simulink model "Check_predictblock"  (R2025b)
settings: Solver=FixedStepAuto  StartTime=0.0  StopTime=1  FixedStep=1/135  RelTol=1e-3
libraries: deeplib x1
settings Model: Creator=faizshaikh  LastModifiedBy=faizshaikh

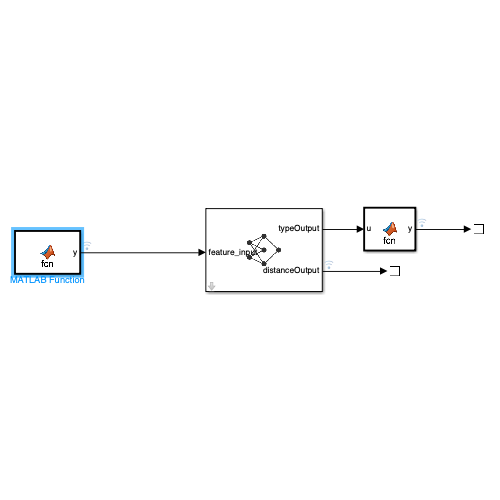
[thumbnail: Simulink's stored preview of the top-level diagram]
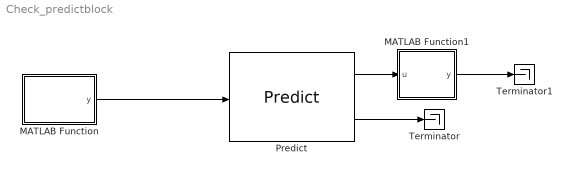
== system Check_predictblock ==
  MATLAB Function : MATLAB Function  TreatAsAtomicUnit=on
  MATLAB Function1 : MATLAB Function  TreatAsAtomicUnit=on
  Predict : deeplib/Predict  Network=Network from MAT-file  NetworkFunction=squeezenet  NetworkFilePath=/Users/faizshaikh/Documents/MATLAB/transmission_system/my_model_test_new.mat  MiniBatchSize=128  InputDataFormats={ 'feature_input', 'CT' }  Predictions=on  Activations={}  ForceInterpretedSim=off  EnableDLNetwork=on  LastKnownNetworkFilePath='/Users/faizshaikh/Documents/MATLAB/transmission_system/my_model_test_new.mat'  LastKnownNetworkTimeStamp=740076.787280092597939074039459228515625
  Terminator : Terminator
  Terminator1 : Terminator
  wires:
  Predict/2 -> Terminator/1
  MATLAB Function/1(y) -> Predict/1
  Predict/1 -> MATLAB Function1/1(u)
  MATLAB Function1/1(y) -> Terminator1/1

== matlab function Check_predictblock/MATLAB Function1 ==
  data: u input; y output
function y = fcn(u)
    [~, winnerIdx] = max(u);
y = winnerIdx;

== matlab function Check_predictblock/MATLAB Function ==
  data: y output
function y = fcn()
    persistent count;

    if isempty(count)
        count = 1; 
    end

    % u is an input port connected to a Counter or Clock
    coder.extrinsic('evalin');
    
    % 1. Pre-define the output 'y' as a 10x321 matrix
    y = zeros(10, 240);
    
    % 2. Pre-define the 3D temporary storage (e.g., for 135 entries)
    % Match the 3rd dimension to your total number of matrices
    data_3D = zeros(10, 321, 135);
    
    % 3. Pull the stacked data
    data_3D = evalin('base', 'DataStack');
    
    % 4. "Loop" by selecting the u-th matrix
    % u should be an integer (1, 2, 3...) coming from a block input
    
    if count <= 135
        y = data_3D(:, 50:289, count);
    else
        y = zeros(10, 240);
    end
    
    count = count + 1;
end
